simulink model "Effectuator"  (R2020a)
settings: Solver=FixedStepDiscrete  StartTime=0.0  StopTime=inf  FixedStep=Ts  RelTol=1e-3
InitFcn:
  | %% Verwende vordefinierte Setpoints (Kreis mit Z-Komponente)
  | 
  | % Config
  | numCircles = 3;
  | scale=6;
  | %Versuch symmetrische Setpunkte zu setzen
  | pointsPerCircle =scale*(4+3*numCircles)+2;
  | 
  | r = 50;
  | m_x = r;
  | m_y = r;
  | 
  | % //
  | s = linspace(0,2*pi,pointsPerCircle);
  | 
  | setPoints_x = [];
  | setPoints_y = [];
  | 
  | for ii=1:numCircles
  | 
  | setPoints_x = [setPoints_x (-cos(s(1:floor(pointsPerCircle / 2))).*r + m_x + 2*r*(ii-1))]; %#ok<AGROW>
  | setPoints_y = [setPoints_y (sin(s).*r+m_y)]; %#ok<AGROW>pointsPerCircle / 2
  | 
  | end
  | 
  | setPoints_x = [setPoints_x flip(setPoints_x(1:end))];
  | 
  | % Loeschen doppelter y-Werte (Kreisuebergang)
  | setPoints_x(pointsPerCircle .* [1:numCircles]) = [];
  | setPoints_y(pointsPerCircle .* [1:numCircles]) = [];
  | 
  | % setPoints_x= [linspace(0,setPoints_x(19),19) setPoints_x(20:end)];
  | % setPoints_y= [linspace(0,setPoints_y(19),19) setPoints_y(20:end)];
  | 
  | % Array Elemente verschieben
  | % setPoints_x = circshift(setPoints_x,-pointsPerCircle/4,2);
  | % setPoints_y = circshift(setPoints_y,-pointsPerCircle/4,2);
  | 
  | z = zeros(1,size(setPoints_x,2));
  | z_x = -5:5;
  | z_y = -z_x.^2 + 25;
  | z_idx = 90;
  | z_idx2 = 210;
  | z(z_idx:z_idx+length(z_x)-1) = z_y;
  | z(z_idx2:z_idx2+length(z_x)-1) = z_y;
  | % z = [z_y z];
  | setPoints_z = z;
  | 
  | % setPoints_x = [zeros(1,length(z_y)) setPoints_x];
  | % setPoints_y = [setPoints_y(1,1)*ones(1,length(z_y)) setPoints_y];
  | 
  | % Umrechnung der Einheiten für Demonstrator
  | % setPoints_x = setPoints_x ./ 1000;
  | % setPoints_y = setPoints_y ./ 1000;
  | % setPoints_z = setPoints_z ./ 1000;
  | 
  | 
  | %{
  | plot(setPoints_x,setPoints_y);
  | fig = figure;
  | plot3(setPoints_x(1:end-1),setPoints_y(1:end-1),setPoints_z(1:end-1));
  | 
  | ax = gca;
  | ax.YDir = 'reverse';
  | ax.ZDir = 'reverse';
  | %}
  | 
  | % setPoints_z = zeros(1,size(setPoints_x,2));
  | 
  | setP_mat = [setPoints_x;setPoints_y;setPoints_z];
  | %Dauerlauftest zehn Durchgänge
  | %setP_mat = repmat(setP_mat, 1, 10);
  | setP_mat = setP_mat(:,2:end);
StartFcn:
  | close all;
model workspace (MAT data in the model file):
  MvmtPerfEval_collectVal = Simulink.Parameter
  MvmtPerfEval_collectVal.Value = 0.65
  MvmtPerfEval_collectVal.Description = '- Anteil eines Interpolationssegments (0,1)
    | - Nach Abarbeitung des spezifizierten Anteils wird gemeinsame Performance aller Agenten
    | vom Dispatcher geladen
    | 
    | - (!!!) Wert MUSS größer sein als MvmtPerfEval_sendOwnVal'
  MvmtPerfEval_collectVal.DataType = 'auto'
  MvmtPerfEval_collectVal.Min = 0
  MvmtPerfEval_collectVal.Max = 1
  MvmtPerfEval_collectVal.Dimensions = [1 1]
  MvmtPerfEval_sendOwnVal = Simulink.Parameter
  MvmtPerfEval_sendOwnVal.Value = 0.6
  MvmtPerfEval_sendOwnVal.Description = '- Anteil eines Interpolationssegments (0,1)
    | - Nach Abarbeitung des spezifizierten Anteils wird Perfomance Kennzahl an Dispatcher übermittelt
    | 
    | - (!!!) Wert MUSS kleiner sein als MvmtPerfEval_collectVal'
  MvmtPerfEval_sendOwnVal.DataType = 'auto'
  MvmtPerfEval_sendOwnVal.Min = 0
  MvmtPerfEval_sendOwnVal.Max = 1
  MvmtPerfEval_sendOwnVal.Dimensions = [1 1]
  PAR_isAxis = Simulink.Parameter
  PAR_isAxis.Value = 1
  PAR_isAxis.DataType = 'auto'
  PAR_isAxis.Dimensions = [1 1]
  PAR_maxVel = Simulink.Parameter
  PAR_maxVel.Value = 5
  PAR_maxVel.DataType = 'auto'
  PAR_maxVel.Dimensions = [1 1]
  PerfEval_numTicks_enable = Simulink.Parameter
  PerfEval_numTicks_enable.Value = 10
  PerfEval_numTicks_enable.Description = 'Anzahl der Ticks (Integrationsschritte), bevor die Performance ausgewertet wird
    | (unabhängig vom Senden des Werts an den Dispatcher)'
  PerfEval_numTicks_enable.DataType = 'auto'
  PerfEval_numTicks_enable.Dimensions = [1 1]
  Segmentregler_I_Gain = Simulink.Parameter
  Segmentregler_I_Gain.Value = 1
  Segmentregler_I_Gain.DataType = 'auto'
  Segmentregler_I_Gain.Dimensions = [1 1]
  Segmentregler_P_Gain = Simulink.Parameter
  Segmentregler_P_Gain.Value = 0
  Segmentregler_P_Gain.DataType = 'auto'
  Segmentregler_P_Gain.Dimensions = [1 1]
  Segmentregler_minVel_enable = Simulink.Parameter
  Segmentregler_minVel_enable.Value = 0.1
  Segmentregler_minVel_enable.DataType = 'auto'
  Segmentregler_minVel_enable.Dimensions = [1 1]
  Segmentregler_numTicks_enable = Simulink.Parameter
  Segmentregler_numTicks_enable.Value = 30
  Segmentregler_numTicks_enable.Description = 'Anzahl der Ticks (Integrationsschritte), bevor der Segmentregler aktiv wird'
  Segmentregler_numTicks_enable.DataType = 'auto'
  Segmentregler_numTicks_enable.Dimensions = [1 1]
  Ts = Simulink.Parameter
  Ts.Value = 0.005
  Ts.Description = 'Sampling Time'
  Ts.DataType = 'auto'
  Ts.Dimensions = [1 1]
  maxPos_x = Simulink.Parameter
  maxPos_x.Value = 300
  maxPos_x.Description = 'Grenze des Arbeitsbereichs (maximaler Wert der Koordinate)'
  maxPos_x.DataType = 'auto'
  maxPos_x.Dimensions = [1 1]
  maxPos_y = Simulink.Parameter
  maxPos_y.Value = 150
  maxPos_y.Description = 'Grenze des Arbeitsbereichs (maximaler Wert der Koordinate)'
  maxPos_y.DataType = 'auto'
  maxPos_y.Dimensions = [1 1]
  maxPos_z = Simulink.Parameter
  maxPos_z.Value = 50
  maxPos_z.Description = 'Grenze des Arbeitsbereichs (maximaler Wert der Koordinate)'
  maxPos_z.DataType = 'auto'
  maxPos_z.Dimensions = [1 1]
  maxVectorLengths = Simulink.Parameter
  maxVectorLengths.Value = 16376
  maxVectorLengths.DataType = 'auto'
  maxVectorLengths.Dimensions = [1 1]
  minAllowedVelSaturation = Simulink.Parameter
  minAllowedVelSaturation.Value = 0.05
  minAllowedVelSaturation.Description = 'Minimaler Saturation-Wert für den Geschwindigkeits-PID-Regler
    | (auch bei Sollgeschwindigkeit soll Fehlerkorrektur möglich sein)'
  minAllowedVelSaturation.DataType = 'auto'
  minAllowedVelSaturation.Dimensions = [1 1]
  numAxes = Simulink.Parameter
  numAxes.Value = 4
  numAxes.DataType = 'auto'
  numAxes.Dimensions = [1 1]
undefined symbols (not defined in the file or in its folder): DiscIntNeverNeededParam
libraries: simulink x6, xpcrtudplib x2, dspnetwork x2, ptplib x1, etargetslib x1, xpcutilitieslib x1
settings Model: xpc_rtwmakecfg_data=_xpcnblib__xpcetherlib__xpcether8255xlib__xpcetherGbElib__xpciplib_  EnablePacing=on  PacingRate=10  Creator=Daniel  LastModifiedBy=Hiwi
settings DataIOCC: ReturnWorkspaceOutputs=off
settings DebuggingCC: AlgebraicLoopMsg=none  ArithmeticOperatorsInVariantConditions=warning
settings SFSimCC: CustomCodeUndefinedFunction=UseInterfaceOnly

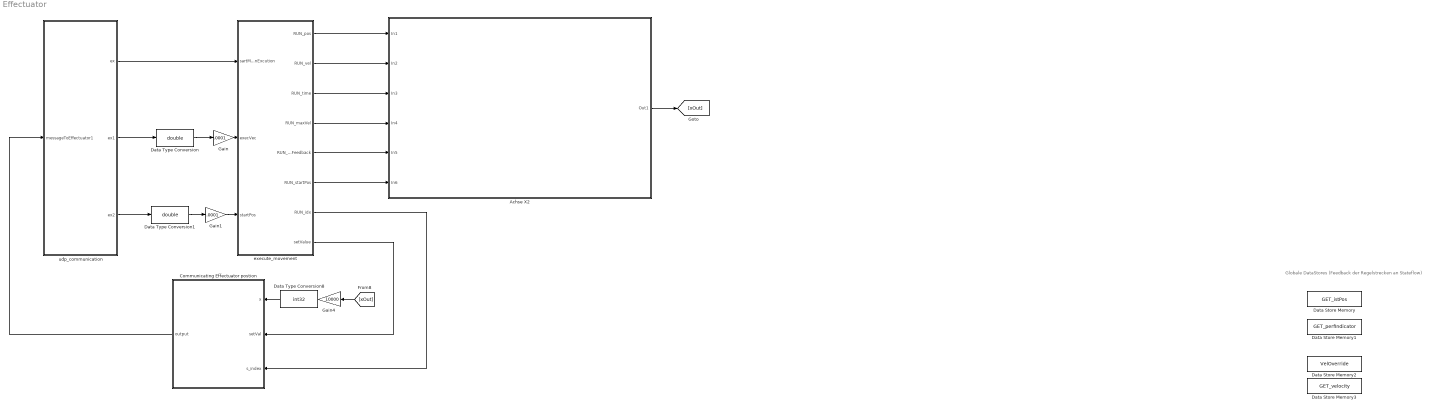
== system Effectuator ==
  note: Globale DataStores (Feedback der Regelstrecken an Stateflow)
  Achse X2 : Subsystem
  Communicating Effectuator postion : MATLAB Function  TreatAsAtomicUnit=on
  Data Store Memory : DataStoreMemory  DataStoreName=GET_istPos  ReadBeforeWriteMsg=warning  WriteAfterWriteMsg=warning  WriteAfterReadMsg=warning  InitialValue=zeros(1,numAxes)  ShowAdditionalParam=off  OutDataTypeStr=double
  Data Store Memory1 : DataStoreMemory  DataStoreName=GET_perfIndicator  ReadBeforeWriteMsg=warning  WriteAfterWriteMsg=warning  WriteAfterReadMsg=warning  InitialValue=zeros(1,numAxes)  ShowAdditionalParam=off  OutDataTypeStr=double
  Data Store Memory2 : DataStoreMemory  DataStoreName=VelOverride  ReadBeforeWriteMsg=warning  WriteAfterWriteMsg=warning  WriteAfterReadMsg=warning  InitialValue=ones(1,numAxes)  ShowAdditionalParam=off  OutDataTypeStr=double
  Data Store Memory3 : DataStoreMemory  DataStoreName=GET_velocity  ReadBeforeWriteMsg=warning  WriteAfterWriteMsg=warning  WriteAfterReadMsg=warning  InitialValue=zeros(1,numAxes)  ShowAdditionalParam=off  OutDataTypeStr=double
  Data Type Conversion : DataTypeConversion  OutDataTypeStr=double
  Data Type Conversion1 : DataTypeConversion  OutDataTypeStr=double
  Data Type Conversion8 : DataTypeConversion  OutDataTypeStr=int32
  Gain : Gain  Gain=.0001
  Gain1 : Gain  Gain=.0001
  Gain4 : Gain  Gain=10000
  execute_movement : Stateflow chart  TreatAsAtomicUnit=on
  udp_communication : Subsystem
  wires:
  udp_communication/2(ex1) -> Data Type Conversion/1
  udp_communication/3(ex2) -> Data Type Conversion1/1
  Data Type Conversion/1 -> Gain/1
  Data Type Conversion1/1 -> Gain1/1
  Achse X2/1(Out1) -> [xOut]
  udp_communication/1(ex) -> execute_movement/1(sartMotionExcution)
  Gain/1 -> execute_movement/2(execVec)
  Gain1/1 -> execute_movement/3(startPos)
  execute_movement/1(RUN_pos) -> Achse X2/1(In1)
  execute_movement/2(RUN_vel) -> Achse X2/2(In2)
  execute_movement/3(RUN_time) -> Achse X2/3(In3)
  execute_movement/4(RUN_maxVel) -> Achse X2/4(In4)
  execute_movement/5(RUN_MvmtPerfFeedback) -> Achse X2/5(In5)
  execute_movement/6(RUN_startPos) -> Achse X2/6(In6)
  Data Type Conversion8/1 -> Communicating Effectuator postion/1(x)
  [xOut] -> Gain4/1
  execute_movement/7(RUN_idx) -> Communicating Effectuator postion/3(s_index)
  Gain4/1 -> Data Type Conversion8/1
  execute_movement/8(setValue) -> Communicating Effectuator postion/2(setVal)
  Communicating Effectuator postion/1(output) -> udp_communication/1(messageToEffectuator1)

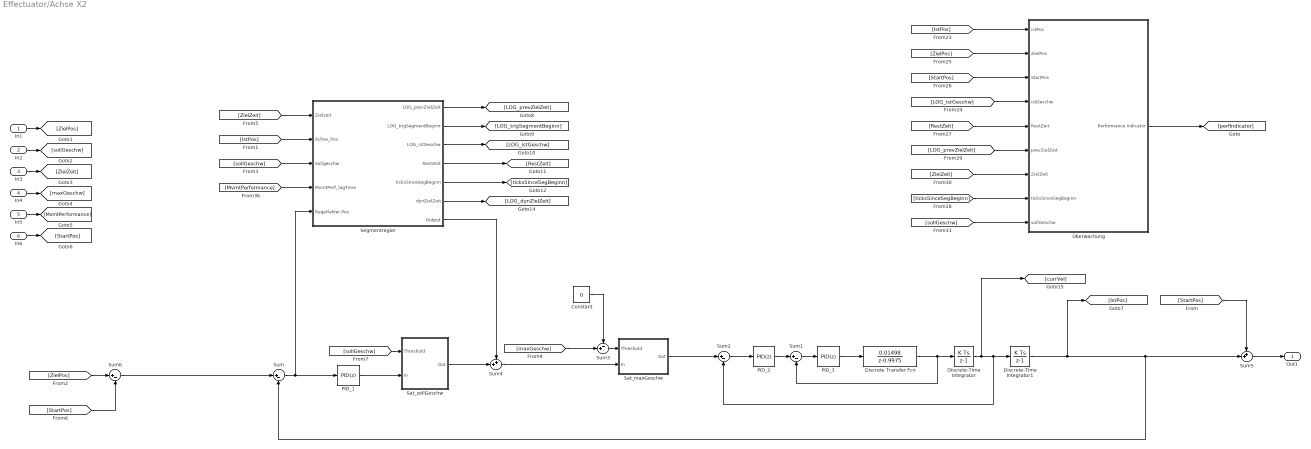
== system Effectuator/Achse X2 ==
  In1 : Inport
  In2 : Inport  Port=2
  In3 : Inport  Port=3
  In4 : Inport  Port=4
  In5 : Inport  Port=5
  In6 : Inport  Port=6
  Constant : Constant  Value=0
  Discrete Transfer Fcn : DiscreteTransferFcn  Numerator=0.01498  Denominator=[1 -0.9975]
  Discrete-Time Integrator : DiscreteIntegrator  SampleTime=-1  ICPrevOutput=DiscIntNeverNeededParam  ICPrevScaledInput=DiscIntNeverNeededParam
  Discrete-Time Integrator1 : DiscreteIntegrator  SampleTime=-1  ICPrevOutput=DiscIntNeverNeededParam  ICPrevScaledInput=DiscIntNeverNeededParam
  PID_1 : simulink/Continuous/PID Controller  Controller=PID  Form=Parallel  TimeDomain=Discrete-time  UseExternalTs=off  SampleTime=-1  IntegratorMethod=Forward Euler  FilterMethod=Forward Euler  ControllerParametersSource=internal  P=20  I=0  D=0  UseFilter=on  N=100  TunerSelectOption=Transfer Function Based (PID Tuner App)  InitialConditionSource=internal  InitialConditionForIntegrator=0  InitialConditionForFilter=0  DifferentiatorICPrevScaledInput=0  ExternalReset=none  TrackingMode=off  Kt=1  LimitOutput=off  UpperSaturationLimit=inf  LowerSaturationLimit=-inf  LinearizeAsGain=off  AntiWindupMode=none  Kb=1  POutMin=[]  POutMax=[]  IOutMin=[]  IOutMax=[]  DOutMin=[]  DOutMax=[]  NOutMin=[]  NOutMax=[]  SumOutMin=[]  SumOutMax=[]  SaturationOutMin=[]  SaturationOutMax=[]  PParamMin=[]  PParamMax=[]  IParamMin=[]  IParamMax=[]  DParamMin=[]  DParamMax=[]  NParamMin=[]  NParamMax=[]  KbParamMin=[]  KbParamMax=[]  KtParamMin=[]  KtParamMax=[]  KbOutMin=[]  KbOutMax=[]  KtOutMin=[]  KtOutMax=[]  IntegratorOutMin=[]  IntegratorOutMax=[]  FilterOutMin=[]  FilterOutMax=[]  SumI1OutMin=[]  SumI1OutMax=[]  SumI2OutMin=[]  SumI2OutMax=[]  SumI3OutMin=[]  SumI3OutMax=[]  SumI4OutMin=[]  SumI4OutMax=[]  SumDOutMin=[]  SumDOutMax=[]  DifferentiatorOutMin=[]  DifferentiatorOutMax=[]  FilterDiffOutCoefMin=[]  FilterDiffOutCoefMax=[]  ReciprocalOutMin=[]  ReciprocalOutMax=[]  SumDenOutMin=[]  SumDenOutMax=[]  SumNumOutMin=[]  SumNumOutMax=[]  DivideOutMin=[]  DivideOutMax=[]  UdiffTsProdOutMin=[]  UdiffTsProdOutMax=[]  NTsProdOutMin=[]  NTsProdOutMax=[]  UintegralTsProdOutMin=[]  UintegralTsProdOutMax=[]  UngainTsProdOutMin=[]  UngainTsProdOutMax=[]  IntegratorContinuousStateAttributes=''  IntegratorStateMustResolveToSignalObject=off  IntegratorRTWStateStorageClass=Auto  FilterContinuousStateAttributes=''  FilterStateMustResolveToSignalObject=off  FilterRTWStateStorageClass=Auto  ParallelPVariant=InternalParameters  IdealPVariant=Disabled  IVariant=InternalParameters  DVariant=InternalParameters  IntegratorVariant=Discrete  SatVariant=Disabled  AWVariant=Passthrough  PCopyVariant=Disabled  TRVariant=Disabled  FdbkBlocksVariant=Forward  IdealPFdbkVariant=Disabled  SatFdbkVariant=Disabled  DerivativeFilterVariant=ForwardEulerFilter  NVariant=InternalParameters  NCopyVariant=Disabled  FilterICVariant=InternalICsFilter  IntegratorICVariant=InternalICs  ExternalResetVariant=Disabled  TRSumVariant=Passthrough  SumFdbkVariant=Disabled  SumVariant=Sum_PID  TsampFilterVariant=InternalTs  TsampNgainVariant=Passthrough  TsampIntegralVariant=Passthrough
  PID_2 : simulink/Continuous/PID Controller  Controller=PID  Form=Parallel  TimeDomain=Discrete-time  UseExternalTs=off  SampleTime=-1  IntegratorMethod=Forward Euler  FilterMethod=Forward Euler  ControllerParametersSource=internal  P=20  I=1  D=0  UseFilter=on  N=100  TunerSelectOption=Transfer Function Based (PID Tuner App)  InitialConditionSource=internal  InitialConditionForIntegrator=0  InitialConditionForFilter=0  DifferentiatorICPrevScaledInput=0  ExternalReset=none  TrackingMode=off  Kt=1  LimitOutput=off  UpperSaturationLimit=inf  LowerSaturationLimit=-inf  LinearizeAsGain=off  AntiWindupMode=none  Kb=1  POutMin=[]  POutMax=[]  IOutMin=[]  IOutMax=[]  DOutMin=[]  DOutMax=[]  NOutMin=[]  NOutMax=[]  SumOutMin=[]  SumOutMax=[]  SaturationOutMin=[]  SaturationOutMax=[]  PParamMin=[]  PParamMax=[]  IParamMin=[]  IParamMax=[]  DParamMin=[]  DParamMax=[]  NParamMin=[]  NParamMax=[]  KbParamMin=[]  KbParamMax=[]  KtParamMin=[]  KtParamMax=[]  KbOutMin=[]  KbOutMax=[]  KtOutMin=[]  KtOutMax=[]  IntegratorOutMin=[]  IntegratorOutMax=[]  FilterOutMin=[]  FilterOutMax=[]  SumI1OutMin=[]  SumI1OutMax=[]  SumI2OutMin=[]  SumI2OutMax=[]  SumI3OutMin=[]  SumI3OutMax=[]  SumI4OutMin=[]  SumI4OutMax=[]  SumDOutMin=[]  SumDOutMax=[]  DifferentiatorOutMin=[]  DifferentiatorOutMax=[]  FilterDiffOutCoefMin=[]  FilterDiffOutCoefMax=[]  ReciprocalOutMin=[]  ReciprocalOutMax=[]  SumDenOutMin=[]  SumDenOutMax=[]  SumNumOutMin=[]  SumNumOutMax=[]  DivideOutMin=[]  DivideOutMax=[]  UdiffTsProdOutMin=[]  UdiffTsProdOutMax=[]  NTsProdOutMin=[]  NTsProdOutMax=[]  UintegralTsProdOutMin=[]  UintegralTsProdOutMax=[]  UngainTsProdOutMin=[]  UngainTsProdOutMax=[]  IntegratorContinuousStateAttributes=''  IntegratorStateMustResolveToSignalObject=off  IntegratorRTWStateStorageClass=Auto  FilterContinuousStateAttributes=''  FilterStateMustResolveToSignalObject=off  FilterRTWStateStorageClass=Auto  ParallelPVariant=InternalParameters  IdealPVariant=Disabled  IVariant=InternalParameters  DVariant=InternalParameters  IntegratorVariant=Discrete  SatVariant=Disabled  AWVariant=Passthrough  PCopyVariant=Disabled  TRVariant=Disabled  FdbkBlocksVariant=Forward  IdealPFdbkVariant=Disabled  SatFdbkVariant=Disabled  DerivativeFilterVariant=ForwardEulerFilter  NVariant=InternalParameters  NCopyVariant=Disabled  FilterICVariant=InternalICsFilter  IntegratorICVariant=InternalICs  ExternalResetVariant=Disabled  TRSumVariant=Passthrough  SumFdbkVariant=Disabled  SumVariant=Sum_PID  TsampFilterVariant=InternalTs  TsampNgainVariant=Passthrough  TsampIntegralVariant=Passthrough
  PID_3 : simulink/Continuous/PID Controller  Controller=PID  Form=Parallel  TimeDomain=Discrete-time  UseExternalTs=off  SampleTime=-1  IntegratorMethod=Forward Euler  FilterMethod=Forward Euler  ControllerParametersSource=internal  P=20  I=1  D=0  UseFilter=on  N=100  TunerSelectOption=Transfer Function Based (PID Tuner App)  InitialConditionSource=internal  InitialConditionForIntegrator=0  InitialConditionForFilter=0  DifferentiatorICPrevScaledInput=0  ExternalReset=none  TrackingMode=off  Kt=1  LimitOutput=off  UpperSaturationLimit=inf  LowerSaturationLimit=-inf  LinearizeAsGain=off  AntiWindupMode=none  Kb=1  POutMin=[]  POutMax=[]  IOutMin=[]  IOutMax=[]  DOutMin=[]  DOutMax=[]  NOutMin=[]  NOutMax=[]  SumOutMin=[]  SumOutMax=[]  SaturationOutMin=[]  SaturationOutMax=[]  PParamMin=[]  PParamMax=[]  IParamMin=[]  IParamMax=[]  DParamMin=[]  DParamMax=[]  NParamMin=[]  NParamMax=[]  KbParamMin=[]  KbParamMax=[]  KtParamMin=[]  KtParamMax=[]  KbOutMin=[]  KbOutMax=[]  KtOutMin=[]  KtOutMax=[]  IntegratorOutMin=[]  IntegratorOutMax=[]  FilterOutMin=[]  FilterOutMax=[]  SumI1OutMin=[]  SumI1OutMax=[]  SumI2OutMin=[]  SumI2OutMax=[]  SumI3OutMin=[]  SumI3OutMax=[]  SumI4OutMin=[]  SumI4OutMax=[]  SumDOutMin=[]  SumDOutMax=[]  DifferentiatorOutMin=[]  DifferentiatorOutMax=[]  FilterDiffOutCoefMin=[]  FilterDiffOutCoefMax=[]  ReciprocalOutMin=[]  ReciprocalOutMax=[]  SumDenOutMin=[]  SumDenOutMax=[]  SumNumOutMin=[]  SumNumOutMax=[]  DivideOutMin=[]  DivideOutMax=[]  UdiffTsProdOutMin=[]  UdiffTsProdOutMax=[]  NTsProdOutMin=[]  NTsProdOutMax=[]  UintegralTsProdOutMin=[]  UintegralTsProdOutMax=[]  UngainTsProdOutMin=[]  UngainTsProdOutMax=[]  IntegratorContinuousStateAttributes=''  IntegratorStateMustResolveToSignalObject=off  IntegratorRTWStateStorageClass=Auto  FilterContinuousStateAttributes=''  FilterStateMustResolveToSignalObject=off  FilterRTWStateStorageClass=Auto  ParallelPVariant=InternalParameters  IdealPVariant=Disabled  IVariant=InternalParameters  DVariant=InternalParameters  IntegratorVariant=Discrete  SatVariant=Disabled  AWVariant=Passthrough  PCopyVariant=Disabled  TRVariant=Disabled  FdbkBlocksVariant=Forward  IdealPFdbkVariant=Disabled  SatFdbkVariant=Disabled  DerivativeFilterVariant=ForwardEulerFilter  NVariant=InternalParameters  NCopyVariant=Disabled  FilterICVariant=InternalICsFilter  IntegratorICVariant=InternalICs  ExternalResetVariant=Disabled  TRSumVariant=Passthrough  SumFdbkVariant=Disabled  SumVariant=Sum_PID  TsampFilterVariant=InternalTs  TsampNgainVariant=Passthrough  TsampIntegralVariant=Passthrough
  Sat_maxGeschw : Subsystem
  Sat_sollGeschw : Subsystem
  Segmentregler : Subsystem
  Sum{,1..2,6} (4 alike) : Sum  Inputs=|+-
  Sum3 : Sum  Inputs=-+|
  Sum4 : Sum  Inputs=++|
  Sum5 : Sum  Inputs=++|
  Überwachung : Subsystem
  Out1 : Outport  VectorParamsAs1DForOutWhenUnconnected=off
  wires:
  Sum/1 -> Segmentregler/5(Regelfehler Pos), PID_1/1
  PID_1/1 -> Sat_sollGeschw/2(In)
  Sat_sollGeschw/1(Out) -> Sum4/2
  Sum4/1 -> Sat_maxGeschw/2(In)
  PID_3/1 -> Discrete Transfer Fcn/1
  Discrete Transfer Fcn/1 -> Discrete-Time Integrator/1, Sum1/2
  Sum2/1 -> PID_2/1
  Sum6/1 -> Sum/1
  Discrete-Time Integrator/1 -> [currVel], Discrete-Time Integrator1/1, Sum2/2
  Sum1/1 -> PID_3/1
  PID_2/1 -> Sum1/1
  Sat_maxGeschw/1(Out) -> Sum2/1
  Discrete-Time Integrator1/1 -> [IstPos], Sum5/2, Sum/2
  Sum5/1 -> Out1/1
  [ZielPos] -> Sum6/1
  [ZielZeit] -> Segmentregler/1(Zielzeit)
  [IstPos] -> Segmentregler/2(Achse_Pos)
  [StartPos] -> Sum5/1
  [StartPos] -> Sum6/2
  [sollGeschw] -> Segmentregler/3(Sollgeschw)
  [sollGeschw] -> Sat_sollGeschw/1(Threshold)
  Segmentregler/1(LOG_prevZielZeit) -> [LOG_prevZielZeit]
  Segmentregler/2(LOG_trigSegmentBeginn) -> [LOG_trigSegmentBeginn]
  Segmentregler/3(LOG_istGeschw) -> [LOG_istGeschw]
  Segmentregler/4(RestZeit) -> [RestZeit]
  [maxGeschw] -> Sum3/2
  Sum3/1 -> Sat_maxGeschw/1(Threshold)
  Constant/1 -> Sum3/1
  [IstPos] -> Überwachung/1(istPos)
  [ZielPos] -> Überwachung/2(ZielPos)
  [StartPos] -> Überwachung/3(StartPos)
  [LOG_istGeschw] -> Überwachung/4(istGeschw)
  [RestZeit] -> Überwachung/5(RestZeit)
  [LOG_prevZielZeit] -> Überwachung/6(prevZielZeit)
  [ZielZeit] -> Überwachung/7(ZielZeit)
  Überwachung/1(Performance Indicator) -> [perfIndicator]
  Segmentregler/5(ticksSinceSegBeginn) -> [ticksSinceSegBeginn]
  [ticksSinceSegBeginn] -> Überwachung/8(ticksSinceSegBeginn)
  [sollGeschw] -> Überwachung/9(sollGeschw)
  [MvmtPerformance] -> Segmentregler/4(MvmtPerf_lagTime)
  Segmentregler/6(dynZielZeit) -> [LOG_dynZielZeit]
  Segmentregler/7(Output) -> Sum4/1
  In1/1 -> [ZielPos]
  In2/1 -> [sollGeschw]
  In4/1 -> [maxGeschw]
  In3/1 -> [ZielZeit]
  In5/1 -> [MvmtPerformance]
  In6/1 -> [StartPos]

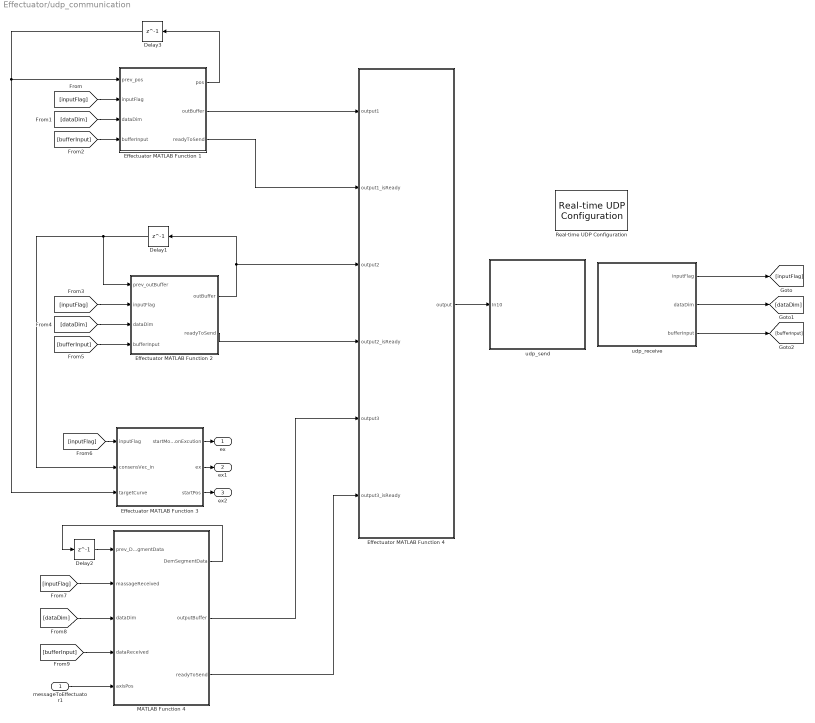
== system Effectuator/udp_communication ==
  messageToEffectuator1 : Inport
  Delay1 : Delay  DelayLength=1
  Delay2 : Delay  DelayLength=1
  Delay3 : Delay  DelayLength=1
  Effectuator MATLAB Function 1 : MATLAB Function  TreatAsAtomicUnit=on
  Effectuator MATLAB Function 2 : MATLAB Function  TreatAsAtomicUnit=on
  Effectuator MATLAB Function 3 : MATLAB Function  TreatAsAtomicUnit=on
  Effectuator MATLAB Function 4 : MATLAB Function  TreatAsAtomicUnit=on
  MATLAB Function 4 : MATLAB Function  TreatAsAtomicUnit=on
  "Real-time UDP Configuration " : ptplib/PTP UDP/Real-time UDP  Configuration   ID=1  IpAddress=192.168.5.100  SubnetMask=255.255.255.0  Gateway=0.0.0.0  EthDrv=Intel Gigabit  PciBus=5  PciSlot=0  PciFunction=0  udpID=0  MulticastList=[]  Multicast={}
      settings: SourceProductBaseCode=XP
  udp_receive : Subsystem
  udp_send : Subsystem
  ex : Outport
  ex1 : Outport  Port=2
  ex2 : Outport  Port=3
  wires:
  udp_receive/3(bufferInput) -> [bufferInput]
  udp_receive/2(dataDim) -> [dataDim]
  udp_receive/1(inputFlag) -> [inputFlag]
  [inputFlag] -> Effectuator MATLAB Function 1/2(inputFlag)
  [dataDim] -> Effectuator MATLAB Function 1/3(dataDim)
  [bufferInput] -> Effectuator MATLAB Function 1/4(bufferInput)
  Delay3/1 -> Effectuator MATLAB Function 1/1(prev_pos), Effectuator MATLAB Function 3/3(targetCurve)
  [dataDim] -> Effectuator MATLAB Function 2/3(dataDim)
  [inputFlag] -> Effectuator MATLAB Function 2/2(inputFlag)
  Delay1/1 -> Effectuator MATLAB Function 2/1(prev_outBuffer), Effectuator MATLAB Function 3/2(consensVec_in)
  [bufferInput] -> Effectuator MATLAB Function 2/4(bufferInput)
  [inputFlag] -> Effectuator MATLAB Function 3/1(inputFlag)
  Effectuator MATLAB Function 1/3(readyToSend) -> Effectuator MATLAB Function 4/2(output1_isReady)
  Effectuator MATLAB Function 2/2(readyToSend) -> Effectuator MATLAB Function 4/4(output2_isReady)
  Effectuator MATLAB Function 4/1(output) -> udp_send/1(In10)
  Effectuator MATLAB Function 1/2(outBuffer) -> Effectuator MATLAB Function 4/1(output1)
  Effectuator MATLAB Function 1/1(pos) -> Delay3/1
  Effectuator MATLAB Function 2/1(outBuffer) -> Delay1/1, Effectuator MATLAB Function 4/3(output2)
  Effectuator MATLAB Function 3/1(startMotionExcution) -> ex/1
  Effectuator MATLAB Function 3/2(ex) -> ex1/1
  Effectuator MATLAB Function 3/3(startPos) -> ex2/1
  MATLAB Function 4/1(DemSegmentData) -> Delay2/1
  Delay2/1 -> MATLAB Function 4/1(prev_DemSegmentData)
  [inputFlag] -> MATLAB Function 4/2(massageReceived)
  [dataDim] -> MATLAB Function 4/3(dataDim)
  [bufferInput] -> MATLAB Function 4/4(dataReceived)
  messageToEffectuator1/1 -> MATLAB Function 4/5(axisPos)
  MATLAB Function 4/2(outputBuffer) -> Effectuator MATLAB Function 4/5(output3)
  MATLAB Function 4/3(readyToSend) -> Effectuator MATLAB Function 4/6(output3_isReady)

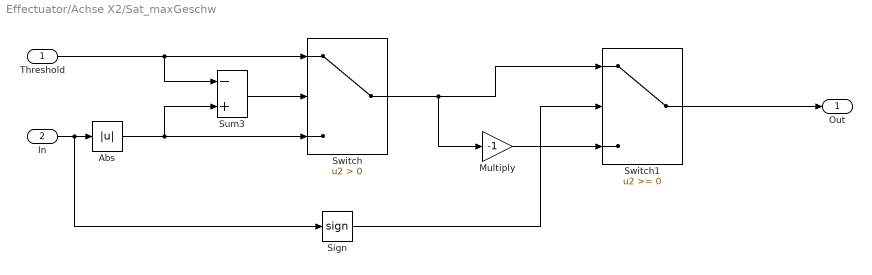
== system Effectuator/Achse X2/Sat_maxGeschw ==
  Threshold : Inport
  In : Inport  Port=2
  Abs : Abs
  Multiply : Gain  Gain=-1
  Sign : Signum
  Sum3 : Sum  Inputs=-+
  Switch : Switch  Criteria=u2 > Threshold
  Switch1 : Switch
  Out : Outport  VectorParamsAs1DForOutWhenUnconnected=off
  wires:
  Switch1/1 -> Out/1
  Multiply/1 -> Switch1/3
  Switch/1 -> Switch1/1, Multiply/1
  Sign/1 -> Switch1/2
  In/1 -> Abs/1, Sign/1
  Abs/1 -> Switch/3, Sum3/2
  Threshold/1 -> Sum3/1, Switch/1
  Sum3/1 -> Switch/2

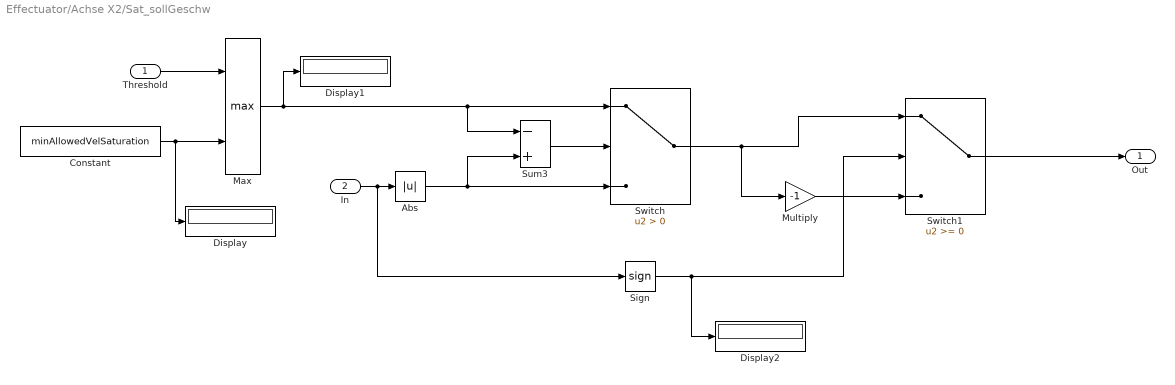
== system Effectuator/Achse X2/Sat_sollGeschw ==
  Threshold : Inport
  In : Inport  Port=2
  Abs : Abs
  Constant : Constant  Value=minAllowedVelSaturation
  Display : Display
  Display1 : Display
  Display2 : Display
  Max : MinMax  Function=max  Inputs=2
  Multiply : Gain  Gain=-1
  Sign : Signum
  Sum3 : Sum  Inputs=-+
  Switch : Switch  Criteria=u2 > Threshold
  Switch1 : Switch
  Out : Outport  VectorParamsAs1DForOutWhenUnconnected=off
  wires:
  Sum3/1 -> Switch/2
  Max/1 -> Display1/1, Switch/1, Sum3/1
  Abs/1 -> Sum3/2, Switch/3
  In/1 -> Sign/1, Abs/1
  Sign/1 -> Display2/1, Switch1/2
  Switch/1 -> Multiply/1, Switch1/1
  Multiply/1 -> Switch1/3
  Switch1/1 -> Out/1
  Threshold/1 -> Max/1
  Constant/1 -> Display/1, Max/2

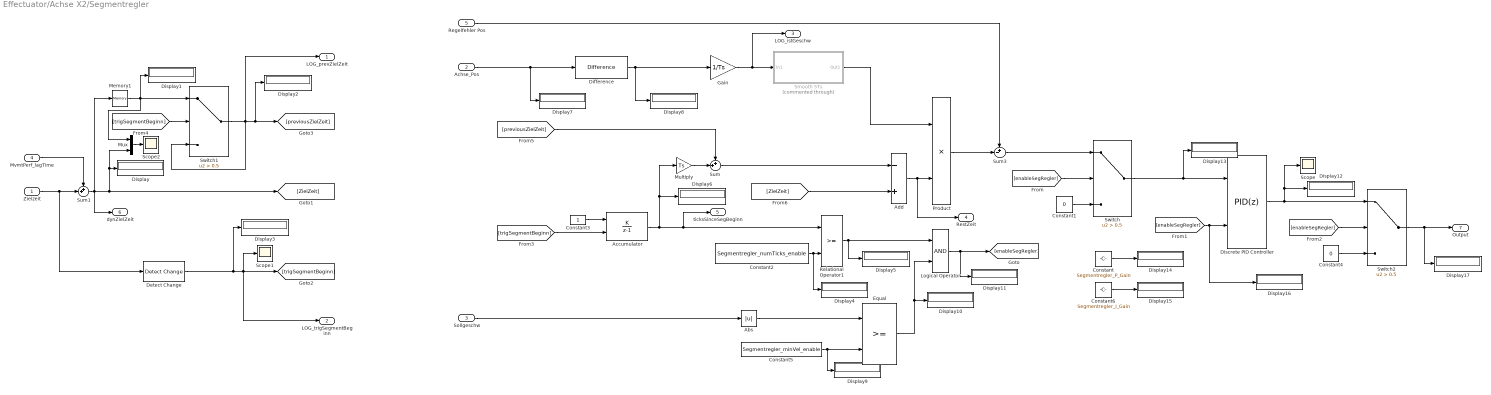
== system Effectuator/Achse X2/Segmentregler ==
  Zielzeit : Inport
  Achse_Pos : Inport  Port=2
  Sollgeschw : Inport  Port=3
  MvmtPerf_lagTime : Inport  Port=4
  Regelfehler Pos : Inport  Port=5
  Abs : Abs
  Accumulator : DiscreteIntegrator  IntegratorMethod=Accumulation: Forward Euler  gainval=1  ExternalReset=rising  SampleTime=-1  ICPrevOutput=DiscIntNeverNeededParam  ICPrevScaledInput=DiscIntNeverNeededParam
  Add : Sum  Inputs=-+
  Constant : Constant  Value=Segmentregler_P_Gain
  Constant1 : Constant  Value=0
  Constant2 : Constant  Value=Segmentregler_numTicks_enable
  Constant3 : Constant
  Constant4 : Constant  Value=0
  Constant5 : Constant  Value=Segmentregler_minVel_enable
  Constant6 : Constant  Value=Segmentregler_I_Gain
  Detect Change : simulink/Logic and Bit Operations/Detect Change  vinit=0  OutDataTypeStr=boolean
  Difference : simulink/Discrete/Difference  ICPrevInput=0.0  OutMin=[]  OutMax=[]  OutDataType=fixdt(1, 16)  OutScaling=2^-10  DoSatur=off
  Discrete PID Controller : simulink/Continuous/PID Controller  Controller=PID  Form=Parallel  TimeDomain=Discrete-time  UseExternalTs=off  SampleTime=-1  IntegratorMethod=Forward Euler  FilterMethod=Forward Euler  ControllerParametersSource=internal  P=Segmentregler_P_Gain  I=Segmentregler_I_Gain  D=0  UseFilter=on  N=100  TunerSelectOption=Transfer Function Based (PID Tuner App)  InitialConditionSource=internal  InitialConditionForIntegrator=0  InitialConditionForFilter=0  DifferentiatorICPrevScaledInput=0  ExternalReset=falling  TrackingMode=off  Kt=1  LimitOutput=off  UpperSaturationLimit=inf  LowerSaturationLimit=-inf  LinearizeAsGain=off  AntiWindupMode=none  Kb=1  POutMin=[]  POutMax=[]  IOutMin=[]  IOutMax=[]  DOutMin=[]  DOutMax=[]  NOutMin=[]  NOutMax=[]  SumOutMin=[]  SumOutMax=[]  SaturationOutMin=[]  SaturationOutMax=[]  PParamMin=[]  PParamMax=[]  IParamMin=[]  IParamMax=[]  DParamMin=[]  DParamMax=[]  NParamMin=[]  NParamMax=[]  KbParamMin=[]  KbParamMax=[]  KtParamMin=[]  KtParamMax=[]  KbOutMin=[]  KbOutMax=[]  KtOutMin=[]  KtOutMax=[]  IntegratorOutMin=[]  IntegratorOutMax=[]  FilterOutMin=[]  FilterOutMax=[]  SumI1OutMin=[]  SumI1OutMax=[]  SumI2OutMin=[]  SumI2OutMax=[]  SumI3OutMin=[]  SumI3OutMax=[]  SumI4OutMin=[]  SumI4OutMax=[]  SumDOutMin=[]  SumDOutMax=[]  DifferentiatorOutMin=[]  DifferentiatorOutMax=[]  FilterDiffOutCoefMin=[]  FilterDiffOutCoefMax=[]  ReciprocalOutMin=[]  ReciprocalOutMax=[]  SumDenOutMin=[]  SumDenOutMax=[]  SumNumOutMin=[]  SumNumOutMax=[]  DivideOutMin=[]  DivideOutMax=[]  UdiffTsProdOutMin=[]  UdiffTsProdOutMax=[]  NTsProdOutMin=[]  NTsProdOutMax=[]  UintegralTsProdOutMin=[]  UintegralTsProdOutMax=[]  UngainTsProdOutMin=[]  UngainTsProdOutMax=[]  IntegratorContinuousStateAttributes=''  IntegratorStateMustResolveToSignalObject=off  IntegratorRTWStateStorageClass=Auto  FilterContinuousStateAttributes=''  FilterStateMustResolveToSignalObject=off  FilterRTWStateStorageClass=Auto  ParallelPVariant=InternalParameters  IdealPVariant=Disabled  IVariant=InternalParameters  DVariant=InternalParameters  IntegratorVariant=Discrete  SatVariant=Disabled  AWVariant=Passthrough  PCopyVariant=Disabled  TRVariant=Disabled  FdbkBlocksVariant=Forward  IdealPFdbkVariant=Disabled  SatFdbkVariant=Disabled  DerivativeFilterVariant=ForwardEulerFilter  NVariant=InternalParameters  NCopyVariant=Disabled  FilterICVariant=InternalICsFilter  IntegratorICVariant=InternalICs  ExternalResetVariant=ExternalReset  TRSumVariant=Passthrough  SumFdbkVariant=Disabled  SumVariant=Sum_PID  TsampFilterVariant=InternalTs  TsampNgainVariant=Passthrough  TsampIntegralVariant=Passthrough
  Display{,1..17} (18 alike) : Display
  Equal : RelationalOperator  OutDataTypeStr=boolean  RndMeth=Simplest
  Gain : Gain  Gain=1/Ts
  Logical Operator : Logic  AllPortsSameDT=off  OutDataTypeStr=boolean
  Memory1 : Memory
  Multiply : Gain  Gain=Ts
  Mux : Mux  Inputs=2
  Product : Product
  Relational Operator1 : RelationalOperator  OutDataTypeStr=boolean  RndMeth=Simplest
  Scope : Scope
  Scope1 : Scope
  Scope2 : Scope
  Smooth 5Ts : Subsystem  Commented=through
  Sum : Sum  Inputs=++|
  Sum1 : Sum  Inputs=++|
  Sum3 : Sum  Inputs=+-|
  Switch : Switch  Criteria=u2 > Threshold  Threshold=0.5
  Switch1 : Switch  Criteria=u2 > Threshold  Threshold=0.5
  Switch2 : Switch  Criteria=u2 > Threshold  Threshold=0.5
  LOG_prevZielZeit : Outport  VectorParamsAs1DForOutWhenUnconnected=off
  LOG_trigSegmentBeginn : Outport  Port=2  VectorParamsAs1DForOutWhenUnconnected=off
  LOG_istGeschw : Outport  Port=3  VectorParamsAs1DForOutWhenUnconnected=off
  RestZeit : Outport  Port=4  VectorParamsAs1DForOutWhenUnconnected=off
  ticksSinceSegBeginn : Outport  Port=5  VectorParamsAs1DForOutWhenUnconnected=off
  dynZielZeit : Outport  Port=6  VectorParamsAs1DForOutWhenUnconnected=off
  Output : Outport  Port=7  VectorParamsAs1DForOutWhenUnconnected=off
  wires:
  Constant3/1 -> Accumulator/1
  Difference/1 -> Display8/1, Gain/1
  Sum3/1 -> Switch/1
  Switch/1 -> Display13/1, Discrete PID Controller/1
  Sum/1 -> Add/1
  Relational Operator1/1 -> Display5/1, Logical Operator/1
  Add/1 -> RestZeit/1, Product/2
  Constant2/1 -> Display4/1, Relational Operator1/2
  Achse_Pos/1 -> Display7/1, Difference/1
  Discrete PID Controller/1 -> Display12/1, Scope/1, Switch2/1
  Constant1/1 -> Switch/3
  Constant4/1 -> Switch2/3
  Product/1 -> Sum3/2
  Regelfehler Pos/1 -> Sum3/1
  Switch2/1 -> Display17/1, Output/1
  Logical Operator/1 -> Display11/1, [enableSegRegler]
  [enableSegRegler] -> Switch/2
  [enableSegRegler] -> Switch2/2
  Sollgeschw/1 -> Abs/1
  Constant5/1 -> Display9/1, Equal/2
  Equal/1 -> Display10/1, Logical Operator/2
  Sum1/1 -> Memory1/1, Mux/2, Display/1, [ZielZeit], dynZielZeit/1
  Gain/1 -> LOG_istGeschw/1, Smooth 5Ts/1(In1)
  Detect Change/1 -> Display3/1, Scope1/1, LOG_trigSegmentBeginn/1, [trigSegmentBeginn]
  [trigSegmentBeginn] -> Switch1/2
  Switch1/1 -> Display2/1, [previousZielZeit], Switch1/3, LOG_prevZielZeit/1
  [previousZielZeit] -> Sum/1
  Smooth 5Ts/1(Out1) -> Product/1
  Multiply/1 -> Sum/2
  [ZielZeit] -> Add/2
  Abs/1 -> Equal/1
  Zielzeit/1 -> Detect Change/1, Sum1/2
  MvmtPerf_lagTime/1 -> Sum1/1
  Accumulator/1 -> Display6/1, Multiply/1, ticksSinceSegBeginn/1, Relational Operator1/1
  [trigSegmentBeginn] -> Accumulator/2
  Constant/1 -> Display14/1
  Constant6/1 -> Display15/1
  [enableSegRegler] -> Display16/1, Discrete PID Controller/2
  Mux/1 -> Scope2/1
  Memory1/1 -> Mux/1, Display1/1, Switch1/1

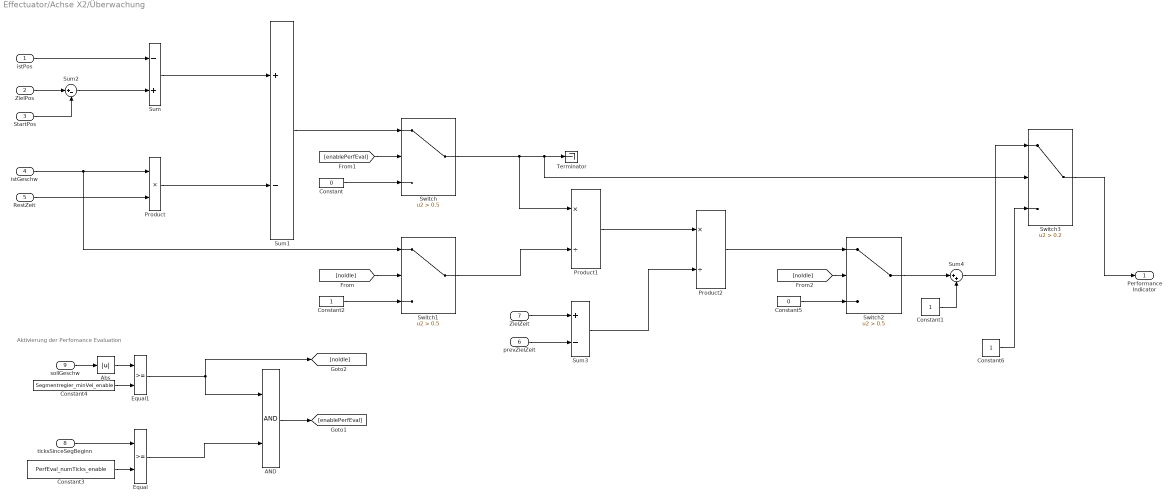
== system Effectuator/Achse X2/Überwachung ==
  note: Aktivierung der Perfomance Evaluation
  istPos : Inport
  ZielPos : Inport  Port=2
  StartPos : Inport  Port=3
  istGeschw : Inport  Port=4
  RestZeit : Inport  Port=5
  prevZielZeit : Inport  Port=6
  ZielZeit : Inport  Port=7
  ticksSinceSegBeginn : Inport  Port=8
  sollGeschw : Inport  Port=9
  AND : Logic  AllPortsSameDT=off  OutDataTypeStr=boolean
  Abs : Abs
  Constant : Constant  Value=0
  Constant1 : Constant
  Constant2 : Constant
  Constant3 : Constant  Value=PerfEval_numTicks_enable
  Constant4 : Constant  Value=Segmentregler_minVel_enable
  Constant5 : Constant  Value=0
  Constant6 : Constant
  Equal : RelationalOperator  OutDataTypeStr=boolean  RndMeth=Simplest
  Equal1 : RelationalOperator  OutDataTypeStr=boolean  RndMeth=Simplest
  Product : Product
  Product1 : Product  Inputs=*/
  Product2 : Product  Inputs=*/
  Sum : Sum  Inputs=-+
  Sum1 : Sum  Inputs=+-
  Sum2 : Sum  Inputs=|+-
  Sum3 : Sum  Inputs=+-
  Sum4 : Sum  Inputs=|++
  Switch : Switch  Criteria=u2 > Threshold  Threshold=0.5
  Switch1 : Switch  Criteria=u2 > Threshold  Threshold=0.5
  Switch2 : Switch  Criteria=u2 > Threshold  Threshold=0.5
  Switch3 : Switch  Criteria=u2 > Threshold  Threshold=0.2
  Terminator : Terminator
  Performance Indicator : Outport  VectorParamsAs1DForOutWhenUnconnected=off
  wires:
  istPos/1 -> Sum/1
  istGeschw/1 -> Switch1/1, Product/1
  RestZeit/1 -> Product/2
  Product/1 -> Sum1/2
  Sum/1 -> Sum1/1
  ZielPos/1 -> Sum2/1
  StartPos/1 -> Sum2/2
  Sum2/1 -> Sum/2
  Sum1/1 -> Switch/1
  Switch/1 -> Product1/1, Switch3/2, Terminator/1
  [enablePerfEval] -> Switch/2
  Constant/1 -> Switch/3
  Product1/1 -> Product2/1
  Sum3/1 -> Product2/2
  prevZielZeit/1 -> Sum3/2
  ZielZeit/1 -> Sum3/1
  Sum4/1 -> Switch3/1
  Constant1/1 -> Sum4/2
  ticksSinceSegBeginn/1 -> Equal/1
  Constant3/1 -> Equal/2
  Equal/1 -> AND/2
  sollGeschw/1 -> Abs/1
  Constant4/1 -> Equal1/2
  Equal1/1 -> [noIdle], AND/1
  AND/1 -> [enablePerfEval]
  [noIdle] -> Switch1/2
  Constant2/1 -> Switch1/3
  Switch1/1 -> Product1/2
  Switch2/1 -> Sum4/1
  Product2/1 -> Switch2/1
  [noIdle] -> Switch2/2
  Constant5/1 -> Switch2/3
  Abs/1 -> Equal1/1
  Switch3/1 -> Performance Indicator/1
  Constant6/1 -> Switch3/3

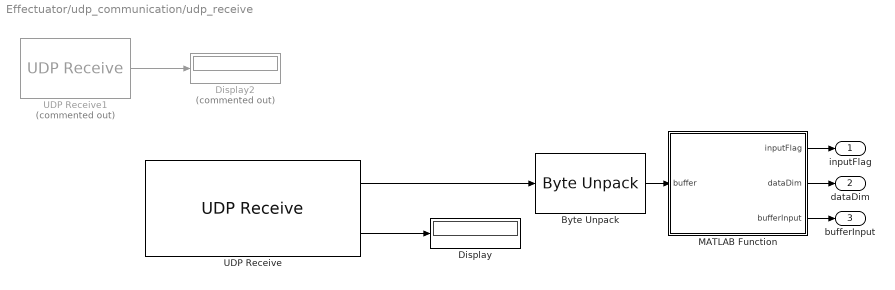
== system Effectuator/udp_communication/udp_receive ==
  Byte Unpack : etargetslib/Byte Unpack  dimensions={[943]}  datatypes={'int32'}  byteAlign=1
  Display : Display
  Display2 : Display  Commented=on
  MATLAB Function : MATLAB Function  TreatAsAtomicUnit=on
  UDP Receive : xpcrtudplib/UDP Receive  ipAddressVal=Use host-target connection  localPort=8080  rcvWidth=943*4  rcvFmAny=off  fmAddress=192.168.5.90  rcvMulticast=off  multicastAddress={}  maxUDPQueue=8  sampleTime=-1
  UDP Receive1 : dspnetwork/UDP Receive  Commented=on  localURL='0.0.0.0'  localPort=8000  remoteURL='192.168.5.90'  remotePort=-1  recvBufferSize=8192  dims=255  signalDatatype=int32  isComplex=off  isVarSize=on  showBlockingTime=on  blockingTime=inf  sampletime=0.01  blockPlatform=HOST
  inputFlag : Outport
  dataDim : Outport  Port=2
  bufferInput : Outport  Port=3
  wires:
  UDP Receive/2 -> Display/1
  UDP Receive/1 -> Byte Unpack/1
  UDP Receive1/1 -> Display2/1
  Byte Unpack/1 -> MATLAB Function/1(buffer)
  MATLAB Function/1(inputFlag) -> inputFlag/1
  MATLAB Function/2(dataDim) -> dataDim/1
  MATLAB Function/3(bufferInput) -> bufferInput/1

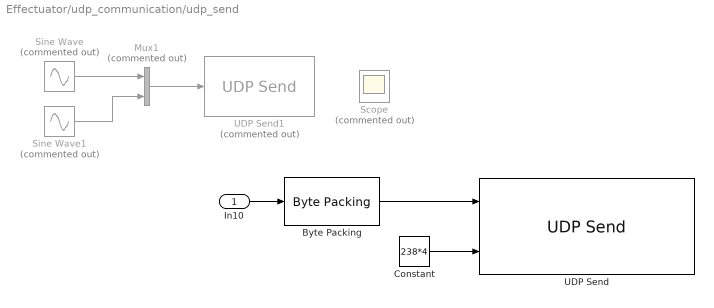
== system Effectuator/udp_communication/udp_send ==
  In10 : Inport
  "Byte Packing " : xpcutilitieslib/Byte Packing   MaskPackedDataType=uint8  MaskUnpackedDataTypes={'int32'}  MaskAlignment=1
  Constant : Constant  Value=238*4
  Mux1 : Mux  Commented=on  Inputs=2
  Scope : Scope  Commented=on
  Sine Wave : Sin  Commented=on  Phase=pi/6  SampleTime=0
  Sine Wave1 : Sin  Commented=on  SampleTime=0
  UDP Send : xpcrtudplib/UDP Send  ipAddressVal=Use host-target connection  localPort=8000  toAddress=192.168.5.90  toPort=8000  sampleTime=-1
      settings: SourceProductBaseCode=XP
  UDP Send1 : dspnetwork/UDP Send  Commented=on  remoteURL='192.168.5.90'  remotePort=8000  localURL='0.0.0.0'  localPortSource=Specify via dialog  localPort=8000  sendBufferSize=8192  sampletime=-1  blockPlatform=HOST  separateLengthPort=0
  wires:
  Constant/1 -> UDP Send/2
  "Byte Packing "/1 -> UDP Send/1
  Mux1/1 -> UDP Send1/1
  Sine Wave/1 -> Mux1/1
  Sine Wave1/1 -> Mux1/2
  In10/1 -> "Byte Packing "/1

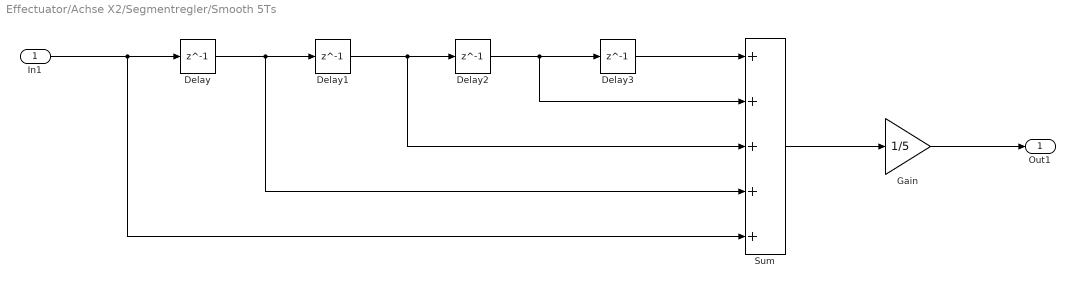
== system Effectuator/Achse X2/Segmentregler/Smooth 5Ts ==
  In1 : Inport
  Delay{,1..3} (4 alike) : Delay  DelayLength=1
  Gain : Gain  Gain=1/5
  Sum : Sum  Inputs=+++++
  Out1 : Outport  VectorParamsAs1DForOutWhenUnconnected=off
  wires:
  In1/1 -> Sum/5, Delay/1
  Delay/1 -> Sum/4, Delay1/1
  Delay1/1 -> Sum/3, Delay2/1
  Delay2/1 -> Sum/2, Delay3/1
  Delay3/1 -> Sum/1
  Sum/1 -> Gain/1
  Gain/1 -> Out1/1

== stateflow chart Effectuator/execute_movement ==
  state Start_Idle
  state Start_run
    entry:
    RUN_idx = 0;
    RUN_startPos = startPos;
    RUN_num_steps = size(execVec,2);
    state Send_command
      entry:
      setValue=1;
      RUN_idx = RUN_idx + 1;
      currStepTimeLength=execVec(3,RUN_idx);
      RUN_pos= execVec(1,RUN_idx);
      RUN_vel = execVec(2,RUN_idx);
      RUN_time = execVec(4,RUN_idx);
      RUN_maxVel = 5;
      RUN_MvmtPerfFeedback= 0;
    state execute_movement
      state idle
        entry:
        setValue=0;
        %waiting for segment excution
      (default) -> idle
    (default) -> Send_command
    (junction 24) -> Send_command
    Send_command -> execute_movement
    execute_movement -> (junction 24) : after(currStepTimeLength,sec)
  (default) -> Start_Idle
  Start_Idle -> Start_run : [sartMotionExcution==1]
  data: sartMotionExcution input; execVec input; startPos input; RUN_pos output; RUN_vel output; RUN_time output; RUN_maxVel output; RUN_MvmtPerfFeedback output; RUN_startPos output; currStepTimeLength local; RUN_num_steps local; RUN_idx output; setValue output int32

== matlab function Effectuator/udp_communication/MATLAB Function 4 ==
  data: prev_DemSegmentData input; DemSegmentData output int32; outputBuffer output int32; massageReceived input int32; dataDim input int32; dataReceived input int32; readyToSend output int32; axisPos input
function [DemSegmentData,outputBuffer,readyToSend]  = fcn(prev_DemSegmentData,massageReceived,dataDim,dataReceived,axisPos)
% UDP Send axes postion
outputBuffer=int32(zeros(1,238));
if(massageReceived==4)
massageSent=int32(3);
outputBuffer(1,1:6) = [int32(massageSent);int32(1);int32(2);axisPos];
outputBuffer(1,6:end)=0;
readyToSend=int32(1);
DemSegmentData=dataReceived(1:7);
else
readyToSend=int32(0);
DemSegmentData=prev_DemSegmentData;
end

== matlab function Effectuator/Communicating Effectuator postion ==
  data: x input; setVal input; output output; s_index input
function output = fcn(x,setVal,s_index)
output=[x;s_index;setVal]

== matlab function Effectuator/udp_communication/udp_receive/MATLAB Function ==
  data: buffer input int32; inputFlag output int32; dataDim output int32; bufferInput output int32
function [inputFlag,dataDim, bufferInput] = fcn(buffer)
inputFlag=buffer(1);
dataDim=[buffer(2) buffer(3)];
bufferInput=(buffer(2:end))';

== matlab function Effectuator/udp_communication/Effectuator MATLAB Function 1 ==
  data: pos output int32; prev_pos input int32; inputFlag input int32; outBuffer output int32; dataDim input int32; bufferInput input int32; readyToSend output int32
function [pos,outBuffer,readyToSend] = fcn(prev_pos,inputFlag,dataDim, bufferInput)
outBuffer=int32(zeros(1,238));

 workspaceCenterX =int32(255);
 workspaceCenterY =int32(50);
 workspaceCenterZ =int32(12.5);
 workspaceWideX =int32(150);
 workspaceWideY =int32(100);
 workspaceWideZ =int32(25);
 startPos =int32(0);
 maxVel =int32(5);

 workspaceXmin = workspaceCenterX - workspaceWideX / 2;
 workspaceXmax = workspaceCenterX + workspaceWideX / 2;
 workspaceYmin = workspaceCenterY - workspaceWideY / 2;
 workspaceYmax = workspaceCenterY + workspaceWideY / 2;
 workspaceZmin = workspaceCenterZ - workspaceWideZ / 2;
 workspaceZmax = workspaceCenterZ + workspaceWideZ / 2;
 
if (inputFlag==1)
 
% get coordination vector
%(1) generate_X2_curve
anzahlSpalten=dataDim(1);
pos=int32(zeros(1,238));
pos(1,1) =int32(1);
pos(1,2) = anzahlSpalten;
x=3;
for  i = 3:anzahlSpalten+2
 if (bufferInput(1,x) >= 1000*workspaceXmin && bufferInput(1,x) <1000*workspaceXmax &&...
				bufferInput(1,x + 1) >= 10000*workspaceYmin && bufferInput(1,x + 1) <=10000*workspaceYmax &&...
				bufferInput(1,x + 2) >=10000* workspaceZmin && bufferInput(1,x + 2) <=1000* workspaceZmax) 
   pos(1,i) = bufferInput(1,x) - 10000*workspaceXmin; 
 else       
			if (i > 2)
				pos(1,i) = pos(1,i - 1);
            else
				pos(1,i) = startPos;
            end
		
 end
end
% generate_koord_vec
anzahlSpalten = pos(1,2);
kooVec=zeros(1,anzahlSpalten + 1);
kooVec(1,1) = int32(1);
kooVec(1,2) = anzahlSpalten - 1;
for i = 3:anzahlSpalten + 1 
    kooVec(1,i) = abs((pos(1,i + 1) - pos(1,i)) / maxVel);
end
outBuffer(1,1:anzahlSpalten +2)=[int32(1) int32(kooVec)];
outBuffer(1,anzahlSpalten +3:end)=int32(0);
readyToSend=int32(1);

else
 pos=prev_pos;
 readyToSend=int32(0);   
end

== matlab function Effectuator/udp_communication/Effectuator MATLAB Function 2 ==
  data: prev_outBuffer input int32; inputFlag input int32; outBuffer output int32; dataDim input int32; bufferInput input int32; readyToSend output int32
function [outBuffer,readyToSend] = fcn(prev_outBuffer,inputFlag,dataDim, bufferInput)
outBuffer=int32(zeros(1,238));
if (inputFlag==2)
anzahlZeilen = bufferInput(1,1);
anzahlSpalten = bufferInput(1,2);
consens=int32(zeros(1,anzahlSpalten + 2));
consens(1,1) = int32(1);
consens(1,2) = anzahlSpalten;
for i = 3: anzahlSpalten + 2
  tMax = bufferInput(1,i);  
  for  j = 1:anzahlZeilen
      if (bufferInput(1,i + j * anzahlSpalten) > tMax)
          tMax = bufferInput(1,i + j * anzahlSpalten);
      end 
  end
  consens(1,i) = tMax;
end
outBuffer(1,1:anzahlSpalten + 3)=[int32(2) int32(consens)];
outBuffer(1,anzahlSpalten + 4:end)=int32(0);
readyToSend=int32(1);

else
 outBuffer=prev_outBuffer;
 readyToSend=int32(0);   
end

== matlab function Effectuator/udp_communication/Effectuator MATLAB Function 3 ==
  data: inputFlag input int32; startMotionExcution output int32; consensVec_in input int32; targetCurve input int32; ex output int32; startPos output int32
function [startMotionExcution,ex,startPos] = fcn(inputFlag,consensVec_in,targetCurve)
consensVec=consensVec_in(1,2:end);
points=int32(zeros(1,235));
speeds=int32(zeros(1,235));
time_periods=int32(zeros(1,235));
absolute_times=int32(zeros(1,235));
ex=int32(zeros(4,235))
startPos=int32(0);
startMotionExcution=int32(0);
% execute_movement
if (inputFlag==3)
startPos=targetCurve(1,3);
points=targetCurve(1,4:end);
speeds=abs(diff(targetCurve(1,3:end)) ./ consensVec(1,3:end));
time_periods=consensVec(1,3:end) ;
absolute_times = cumsum(consensVec(1,3:end));   
ex=[points;speeds;time_periods;absolute_times];   
startMotionExcution=int32(1);
else 
 startMotionExcution=int32(0);
end

== matlab function Effectuator/udp_communication/Effectuator MATLAB Function 4 ==
  data: output1 input int32; output1_isReady input int32; output output int32 size=[1 238]; output2 input int32; output2_isReady input int32; output3 input; output3_isReady input
function output = fcn(output1,output1_isReady,output2,output2_isReady,output3,output3_isReady)
output = int32(zeros(1,238));
if (output1_isReady==1)
  output=output1;
elseif(output2_isReady==1)
  output=output2;
else(output3_isReady==1)
  output=output3;  
end
